simulink model "gm_DSBF"  (R2019b)
settings: Solver=FixedStepDiscrete  StartTime=0.0  StopTime=0.02  RelTol=1e-3
InitFcn:
  | sm_callback_init
StopFcn:
  | sm_callback_stop
undefined symbols (not defined in the file or in its folder): arraySize, arraySpacing, delayDataTypeFractionLength, delayDataTypeSign, delayDataTypeWordLength, mp, samplingRate, speedOfSound, upsampleFactor
libraries: hdlsllib x64, simulink x36, dspmlti4 x16, dsphdlfiltering x16
(part 1 of 5)
settings Model: Creator=Ross  LastModifiedBy=tyler
settings DataIOCC: ReturnWorkspaceOutputs=off
settings OptimizationCC: BlockReduction=off  ConditionallyExecuteInputs=off  DefaultParameterBehavior=Inlined
settings DebuggingCC: ReadBeforeWriteMsg=DisableAll  WriteAfterWriteMsg=DisableAll  WriteAfterReadMsg=DisableAll  AlgebraicLoopMsg=error  InheritedTsInSrcMsg=none  MultiTaskDSMMsg=none  SingleTaskRateTransMsg=error  PregeneratedLibrarySubsystemCodeDiagnostic=none  ArithmeticOperatorsInVariantConditions=warning
settings HardwareCC: ProdBitPerPointer=32  ProdBitPerSizeT=32  ProdBitPerPtrDiffT=32  ProdLargestAtomicFloat=None  ProdIntDivRoundTo=Undefined  ProdEndianess=Unspecified  ProdWordSize=32  ProdHWDeviceType=ASIC/FPGA->ASIC/FPGA  TargetBitPerPointer=64  TargetBitPerSizeT=64  TargetBitPerPtrDiffT=64  TargetLongLongMode=on  TargetIntDivRoundTo=Zero  TargetEndianess=LittleEndian  TargetWordSize=64  TargetHWDeviceType=Custom Processor->MATLAB Host Computer  ProdEqTarget=off
settings ModelReferenceCC: UpdateModelReferenceTargets=IfOutOfDate
settings SFSimCC: SFSimEcho=off  SimUseLocalCustomCode=off  CustomCodeUndefinedFunction=UseInterfaceOnly
settings RTWCC: RTWUseLocalCustomCode=off

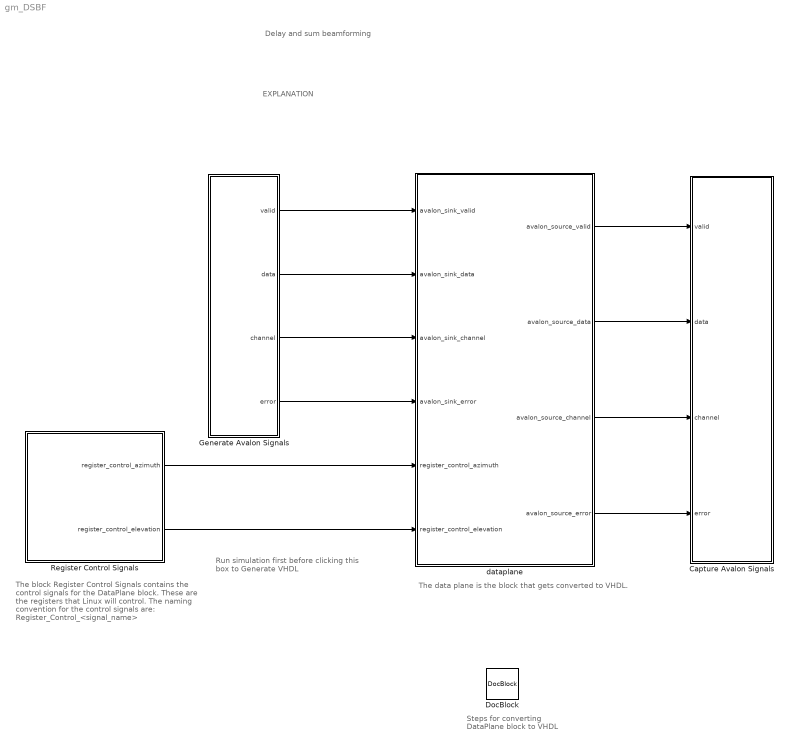
== system gm_DSBF ==
  note: The block Register Control Signals contains
      | the control signals for the DataPlane block.
      | These are the registers that Linux will control.
      | The naming convention for the control
      | signals are:  Register_Control_<signal_name>
  note: Run simulation first
      | before clicking this box to
      | Generate VHDL
  note: Delay and sum beamforming
  note: Steps for converting
      | DataPlane block
      | to VHDL
  note: EXPLANATION
  note: The data plane is the block that gets converted to VHDL.
  Capture Avalon Signals : Subsystem
  DocBlock : simulink/Model-Wide Utilities/DocBlock  DocumentType=HTML
  Generate Avalon Signals : Subsystem
  Register Control Signals : Subsystem
  dataplane : Subsystem  TreatAsAtomicUnit=on
  wires:
  Register Control Signals/2(register_control_elevation) -> dataplane/6(register_control_elevation)
  Register Control Signals/1(register_control_azimuth) -> dataplane/5(register_control_azimuth)
  dataplane/4(avalon_source_error) -> Capture Avalon Signals/4(error)
  dataplane/3(avalon_source_channel) -> Capture Avalon Signals/3(channel)
  dataplane/1(avalon_source_valid) -> Capture Avalon Signals/1(valid)
  dataplane/2(avalon_source_data) -> Capture Avalon Signals/2(data)
  Generate Avalon Signals/4(error) -> dataplane/4(avalon_sink_error)
  Generate Avalon Signals/3(channel) -> dataplane/3(avalon_sink_channel)
  Generate Avalon Signals/1(valid) -> dataplane/1(avalon_sink_valid)
  Generate Avalon Signals/2(data) -> dataplane/2(avalon_sink_data)

== system gm_DSBF/Capture Avalon Signals ==
  note: Note:  If these "To Workspace" variables show up under a variable called "out",
      | Open the Configure Logging... window (Simulation->Output->Configure Logging...)
      | and deselect the checkbox "Single simulation output:" found under the "Save to workspace or file" section.
  valid : Inport
  data : Inport  Port=2
  channel : Inport  Port=3
  error : Inport  Port=4
  To Workspace : ToWorkspace  VariableName=Avalon_Sink_Data  SaveFormat=Timeseries  SampleTime=-1
  To Workspace1 : ToWorkspace  VariableName=Avalon_Sink_Valid  SaveFormat=Timeseries  SampleTime=-1
  To Workspace2 : ToWorkspace  VariableName=Avalon_Sink_Channel  SaveFormat=Timeseries  SampleTime=-1
  To Workspace3 : ToWorkspace  VariableName=Avalon_Sink_Error  SaveFormat=Timeseries  SampleTime=-1
  wires:
  channel/1 -> To Workspace2/1
  error/1 -> To Workspace3/1
  valid/1 -> To Workspace1/1
  data/1 -> To Workspace/1

== system gm_DSBF/Generate Avalon Signals ==
  note: Avalon Streaming Sink Signals
      | Note: We are assuming a specific system clock frequency that these signals are being clock in at.
      | The interface needs to be regenerated if this system clock frequency changes. Change system clock frequency in InitFcn callback in Model Explorer.
      |
      | -- Avalon streaming slave interface (sink)
      | AD1939_DAC_data : in std_logic_vector(31 downto 0); -- W=32; F=28; Signed 2's Complement
      | AD1939_DAC_channel : in std_logic_vector(1 downto 0); -- Left <-> channel 0; Right <-> channel 1 (other two channels are ignored)
      | AD1939_DAC_valid : in std_logic; -- asserted when data is valid
      | AD1939_DAC_error : in std_logic_vector(1 downto 0) -- error channel is ignored, assumed to be error free at this point
      |
      | For more information on the data-channel-valid protocol, see chapter 5 in Intel's Avalon Interfaced Specification (p. 40) at https://www.intel.com/content/dam/www/programmable/us/en/pdfs/literature/manual/mnl_avalon_spec.pdf
  Avalon Source Channel : FromWorkspace  VariableName=mp.Avalon_Source_Channel  OutDataTypeStr=double  SampleTime=mp.Ts_system
  "Avalon Source Data " : FromWorkspace  VariableName=mp.Avalon_Source_Data  OutDataTypeStr=double  SampleTime=mp.Ts_system
  Avalon Source Error : FromWorkspace  VariableName=mp.Avalon_Source_Error  OutDataTypeStr=double  SampleTime=mp.Ts_system
  Avalon Source Valid : FromWorkspace  VariableName=mp.Avalon_Source_Valid  OutDataTypeStr=double  SampleTime=mp.Ts_system
  Data Type Conversion : DataTypeConversion  OutDataTypeStr=fixdt(1,mp.W_bits,mp.F_bits)
  Data Type Conversion1 : DataTypeConversion  OutDataTypeStr=fixdt(0,4,0)
  Data Type Conversion2 : DataTypeConversion  OutDataTypeStr=boolean
  Data Type Conversion3 : DataTypeConversion  OutDataTypeStr=fixdt(0,2,0)
  valid : Outport  VectorParamsAs1DForOutWhenUnconnected=off
  data : Outport  Port=2  VectorParamsAs1DForOutWhenUnconnected=off
  channel : Outport  Port=3  VectorParamsAs1DForOutWhenUnconnected=off
  error : Outport  Port=4  VectorParamsAs1DForOutWhenUnconnected=off
  wires:
  "Avalon Source Data "/1 -> Data Type Conversion/1
  Avalon Source Channel/1 -> Data Type Conversion1/1
  Data Type Conversion3/1 -> error/1
  Avalon Source Valid/1 -> Data Type Conversion2/1
  Data Type Conversion/1 -> data/1
  Avalon Source Error/1 -> Data Type Conversion3/1
  Data Type Conversion2/1 -> valid/1
  Data Type Conversion1/1 -> channel/1

== system gm_DSBF/Register Control Signals ==
  note: Control Signals that will be coming from Linux via
      | memory mapped registers need to have names
      | containing the prefix "register_control_"
      | (all lower case)
  Data Type Conversion1 : DataTypeConversion  OutDataTypeStr=mp.register(2).dataType
  Data Type Conversion2 : DataTypeConversion  OutDataTypeStr=mp.register(1).dataType
  Time Series Signal from Workspace 1 : FromWorkspace  VariableName=mp.register(1).timeseries  OutDataTypeStr=double  SampleTime=mp.Ts_system
  Time Series Signal from Workspace 2 : FromWorkspace  VariableName=mp.register(2).timeseries  OutDataTypeStr=double  SampleTime=mp.Ts_system
  register_control_azimuth : Outport  VectorParamsAs1DForOutWhenUnconnected=off
  register_control_elevation : Outport  Port=2  VectorParamsAs1DForOutWhenUnconnected=off
  wires:
  Data Type Conversion1/1 -> register_control_elevation/1
  Data Type Conversion2/1 -> register_control_azimuth/1
  Time Series Signal from Workspace 2/1 -> Data Type Conversion1/1
  Time Series Signal from Workspace 1/1 -> Data Type Conversion2/1

== system gm_DSBF/dataplane ==
  avalon_sink_valid : Inport  OutDataTypeStr=boolean  PortDimensions=1  SampleTime=1.01725260416667e-08
  avalon_sink_data : Inport  Port=2  OutDataTypeStr=fixdt(1, 32, 28)  PortDimensions=1  SampleTime=1.01725260416667e-08
  avalon_sink_channel : Inport  Port=3  OutDataTypeStr=fixdt(0, 4, 0)  PortDimensions=1  SampleTime=1.01725260416667e-08
  avalon_sink_error : Inport  Port=4  OutDataTypeStr=fixdt(0, 2, 0)  PortDimensions=1  SampleTime=1.01725260416667e-08
  register_control_azimuth : Inport  Port=5  OutDataTypeStr=fixdt(1, 16, 8)  PortDimensions=1  SampleTime=1.01725260416667e-08
  register_control_elevation : Inport  Port=6  OutDataTypeStr=fixdt(1, 16, 8)  PortDimensions=1  SampleTime=1.01725260416667e-08
  Avalon Data Processing : Subsystem
  Delay{,1..3} (4 alike) : Delay  DelayLength=double(1)  InitialCondition=0  SampleTime=1.01725260416667e-08
  compute projections : Subsystem
  compute_delays : Subsystem
  delayMatch : Delay  DelayLength=double(6144)  InitialCondition=0  SampleTime=1.01725260416667e-08
  delayMatch1 : Delay  DelayLength=double(6144)  InitialCondition=0  SampleTime=1.01725260416667e-08
  avalon_source_valid : Outport  VectorParamsAs1DForOutWhenUnconnected=off
  avalon_source_data : Outport  Port=2  VectorParamsAs1DForOutWhenUnconnected=off
  avalon_source_channel : Outport  Port=3  VectorParamsAs1DForOutWhenUnconnected=off
  avalon_source_error : Outport  Port=4  VectorParamsAs1DForOutWhenUnconnected=off
  wires:
  avalon_sink_valid/1 -> Avalon Data Processing/1(valid_in)
  avalon_sink_data/1 -> Avalon Data Processing/2(Sink_Data)
  avalon_sink_channel/1 -> Avalon Data Processing/3(Sink_Channel)
  delayMatch1/1 -> avalon_source_error/1
  register_control_azimuth/1 -> compute projections/1(azimuth)
  register_control_elevation/1 -> compute projections/2(elevation)
  Avalon Data Processing/1(Source_Data) -> avalon_source_data/1
  delayMatch/1 -> avalon_source_channel/1
  Avalon Data Processing/3(Source_Valid) -> avalon_source_valid/1
  Delay/1 -> compute_delays/3(sin_elevation)
  Delay1/1 -> compute_delays/2(cos_elevation)
  Delay2/1 -> compute_delays/1(sin_azimuth)
  Delay3/1 -> Avalon Data Processing/4(delays)
  compute projections/1(sin_azimuth) -> Delay2/1
  compute projections/2(cos_elevation) -> Delay1/1
  compute projections/3(sin_elevation) -> Delay/1
  compute_delays/1(delays) -> Delay3/1
  Avalon Data Processing/2(Source_Channel) -> delayMatch/1
  avalon_sink_error/1 -> delayMatch1/1

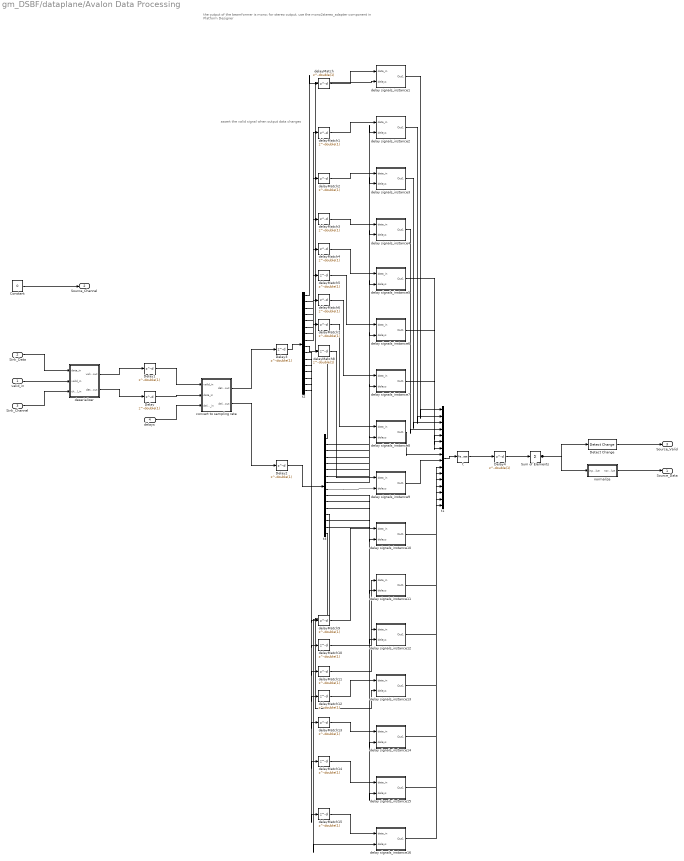
== system gm_DSBF/dataplane/Avalon Data Processing ==
  note: the output of the beamformer is mono; for stereo output, use the mono2stereo_adapter component in Platform Designer
  note: assert the valid signal when output data changes
  valid_in : Inport  OutDataTypeStr=boolean  PortDimensions=1  SampleTime=1.01725260416667e-08
  Sink_Data : Inport  Port=2  OutDataTypeStr=fixdt(1, 32, 28)  PortDimensions=1  SampleTime=1.01725260416667e-08
  Sink_Channel : Inport  Port=3  OutDataTypeStr=fixdt(0, 4, 0)  PortDimensions=1  SampleTime=1.01725260416667e-08
  delays : Inport  Port=4  OutDataTypeStr=fixdt(1, 12, 6)  PortDimensions=[16]  SampleTime=1.01725260416667e-08
  Constant : Constant  Value=0  OutDataTypeStr=fixdt(0, 1, 0)  SampleTime=-1
  Delay : Delay  DelayLength=double(1)  InitialCondition=0  SampleTime=1.01725260416667e-08
  Delay1 : Delay  DelayLength=double(1)  InitialCondition=0  SampleTime=1.01725260416667e-08
  Delay2 : Delay  DelayLength=double(1)  InitialCondition=0  SampleTime=2.08333333333333e-05
  Delay3 : Delay  DelayLength=double(1)  InitialCondition=0  SampleTime=2.08333333333333e-05
  Delay4 : Delay  DelayLength=double(1)  InitialCondition=0  SampleTime=1.01725260416667e-08
  Detect Change : simulink/Logic and Bit Operations/Detect Change  vinit=0  OutDataTypeStr=boolean
  Sum of Elements : Sum  Inputs=+  AccumDataTypeStr=fixdt(1, 36, 28)  OutDataTypeStr=fixdt(1, 36, 28)  SampleTime=1.01725260416667e-08
  convert to sampling rate : Subsystem
  delay signals_instance1 : Subsystem
  delay signals_instance10 : Subsystem
  delay signals_instance11 : Subsystem
  delay signals_instance12 : Subsystem
  delay signals_instance13 : Subsystem
  delay signals_instance14 : Subsystem
  delay signals_instance15 : Subsystem
  delay signals_instance16 : Subsystem
  delay signals_instance2 : Subsystem
  delay signals_instance3 : Subsystem
  delay signals_instance4 : Subsystem
  delay signals_instance5 : Subsystem
  delay signals_instance6 : Subsystem
  delay signals_instance7 : Subsystem
  delay signals_instance8 : Subsystem
  delay signals_instance9 : Subsystem
  delayMatch{,1..15} (16 alike) : Delay  DelayLength=double(1)  InitialCondition=0  SampleTime=2.08333333333333e-05
  deserializer : Subsystem
  normalize : Subsystem
  t : Reshape
  t1 : Concatenate  NumInputs=16
  t2 : Demux  Outputs=16
  t3 : Demux  Outputs=16
  Source_Data : Outport  InitialOutput=0  VectorParamsAs1DForOutWhenUnconnected=off
  Source_Channel : Outport  Port=2  InitialOutput=0  VectorParamsAs1DForOutWhenUnconnected=off
  Source_Valid : Outport  Port=3  InitialOutput=0  VectorParamsAs1DForOutWhenUnconnected=off
  wires:
  Delay/1 -> convert to sampling rate/2(data_in)
  Delay1/1 -> convert to sampling rate/1(valid_in)
  Delay2/1 -> t3/1
  Delay3/1 -> t2/1
  Delay4/1 -> Sum of Elements/1
  Detect Change/1 -> Source_Valid/1
  Sum of Elements/1 -> Detect Change/1, normalize/1(input_value)
  convert to sampling rate/1(data_out) -> Delay3/1
  convert to sampling rate/2(delays_out) -> Delay2/1
  t/1 -> Delay4/1
  deserializer/1(valid_out) -> Delay1/1
  deserializer/2(data_out) -> Delay/1
  delay signals_instance1/1(Out1) -> t1/1
  delay signals_instance2/1(Out1) -> t1/2
  delay signals_instance3/1(Out1) -> t1/3
  delay signals_instance4/1(Out1) -> t1/4
  delay signals_instance5/1(Out1) -> t1/5
  delay signals_instance6/1(Out1) -> t1/6
  delay signals_instance7/1(Out1) -> t1/7
  delay signals_instance8/1(Out1) -> t1/8
  delay signals_instance9/1(Out1) -> t1/9
  delay signals_instance10/1(Out1) -> t1/10
  delay signals_instance11/1(Out1) -> t1/11
  delay signals_instance12/1(Out1) -> t1/12
  delay signals_instance13/1(Out1) -> t1/13
  delay signals_instance14/1(Out1) -> t1/14
  delay signals_instance15/1(Out1) -> t1/15
  delay signals_instance16/1(Out1) -> t1/16
  normalize/1(normalized_value) -> Source_Data/1
  Constant/1 -> Source_Channel/1
  delayMatch/1 -> delay signals_instance1/1(data_in)
  delayMatch1/1 -> delay signals_instance2/1(data_in)
  delayMatch2/1 -> delay signals_instance3/1(data_in)
  delayMatch3/1 -> delay signals_instance4/1(data_in)
  delayMatch4/1 -> delay signals_instance5/1(data_in)
  delayMatch5/1 -> delay signals_instance6/1(data_in)
  delayMatch6/1 -> delay signals_instance7/1(data_in)
  delayMatch7/1 -> delay signals_instance8/1(data_in)
  delayMatch8/1 -> delay signals_instance9/1(data_in)
  delayMatch9/1 -> delay signals_instance10/1(data_in)
  delayMatch10/1 -> delay signals_instance11/1(data_in)
  delayMatch11/1 -> delay signals_instance12/1(data_in)
  delayMatch12/1 -> delay signals_instance13/1(data_in)
  delayMatch13/1 -> delay signals_instance14/1(data_in)
  delayMatch14/1 -> delay signals_instance15/1(data_in)
  delayMatch15/1 -> delay signals_instance16/1(data_in)
  t3/1 -> delay signals_instance1/2(delays)
  t3/2 -> delay signals_instance2/2(delays)
  t3/3 -> delay signals_instance3/2(delays)
  t3/4 -> delay signals_instance4/2(delays)
  t3/5 -> delay signals_instance5/2(delays)
  t3/6 -> delay signals_instance6/2(delays)
  t3/7 -> delay signals_instance7/2(delays)
  t3/8 -> delay signals_instance8/2(delays)
  t3/9 -> delay signals_instance9/2(delays)
  t3/10 -> delay signals_instance10/2(delays)
  t3/11 -> delay signals_instance11/2(delays)
  t3/12 -> delay signals_instance12/2(delays)
  t3/13 -> delay signals_instance13/2(delays)
  t3/14 -> delay signals_instance14/2(delays)
  t3/15 -> delay signals_instance15/2(delays)
  t3/16 -> delay signals_instance16/2(delays)
  t1/1 -> t/1
  valid_in/1 -> deserializer/2(valid_in)
  Sink_Data/1 -> deserializer/1(data_in)
  Sink_Channel/1 -> deserializer/3(channel_in)
  delays/1 -> convert to sampling rate/3(delays_in)
  t2/1 -> delayMatch/1
  t2/2 -> delayMatch1/1
  t2/3 -> delayMatch2/1
  t2/4 -> delayMatch3/1
  t2/5 -> delayMatch4/1
  t2/6 -> delayMatch5/1
  t2/7 -> delayMatch6/1
  t2/8 -> delayMatch7/1
  t2/9 -> delayMatch8/1
  t2/10 -> delayMatch9/1
  t2/11 -> delayMatch10/1
  t2/12 -> delayMatch11/1
  t2/13 -> delayMatch12/1
  t2/14 -> delayMatch13/1
  t2/15 -> delayMatch14/1
  t2/16 -> delayMatch15/1

== system gm_DSBF/dataplane/compute projections ==
  azimuth : Inport  OutDataTypeStr=fixdt(1, 16, 8)  PortDimensions=1  SampleTime=1.01725260416667e-08
  elevation : Inport  Port=2  OutDataTypeStr=fixdt(1, 16, 8)  PortDimensions=1  SampleTime=1.01725260416667e-08
  compute cosine : Subsystem
  compute sine : Subsystem
  compute sine1 : Subsystem
  sin_azimuth : Outport
  cos_elevation : Outport  Port=2
  sin_elevation : Outport  Port=3
  wires:
  compute cosine/1(Out1) -> cos_elevation/1
  compute sine/1(output_value) -> sin_azimuth/1
  compute sine1/1(output_value) -> sin_elevation/1
  azimuth/1 -> compute sine/1(angle)
  elevation/1 -> compute sine1/1(angle), compute cosine/1(angle)

== system gm_DSBF/dataplane/compute_delays ==
  sin_azimuth : Inport  OutDataTypeStr=fixdt(1, 16, 14)  PortDimensions=1  SampleTime=1.01725260416667e-08
  cos_elevation : Inport  Port=2  OutDataTypeStr=fixdt(1, 16, 14)  PortDimensions=1  SampleTime=1.01725260416667e-08
  sin_elevation : Inport  Port=3  OutDataTypeStr=fixdt(1, 16, 14)  PortDimensions=1  SampleTime=1.01725260416667e-08
  compute_delays : MATLAB Function  TreatAsAtomicUnit=on
  delayMatch : Delay  DelayLength=double(4)  InitialCondition=0  SampleTime=1.01725260416667e-08
  delays : Outport  VectorParamsAs1DForOutWhenUnconnected=off
  wires:
  delayMatch/1 -> compute_delays/2(cos_elevation)
  compute_delays/1(delays) -> delays/1
  sin_azimuth/1 -> compute_delays/1(sin_azimuth)
  cos_elevation/1 -> delayMatch/1
  sin_elevation/1 -> compute_delays/3(sin_elevation)

== system gm_DSBF/dataplane/Avalon Data Processing/convert to sampling rate ==
  note: sample and data on the valid pulse to make sure we are only using valid data
  valid_in : Inport  OutDataTypeStr=boolean  PortDimensions=1  SampleTime=1.01725260416667e-08
  data_in : Inport  Port=2  OutDataTypeStr=fixdt(1, 32, 28)  PortDimensions=[16]  SampleTime=1.01725260416667e-08
  delays_in : Inport  Port=3  OutDataTypeStr=fixdt(1, 12, 6)  PortDimensions=[16]  SampleTime=1.01725260416667e-08
  PipelineRegister : Delay  DelayLength=double(1)  InitialCondition=0  SampleTime=2.08333333333333e-05
  PipelineRegister1 : Delay  DelayLength=double(1)  InitialCondition=0  SampleTime=2.08333333333333e-05
  Rate Transition1 : RateTransition  InitialCondition=double(0)  OutPortSampleTimeOpt=Multiple of input port sample time  OutPortSampleTimeMultiple=2048
  Rate Transition2 : DownSample  N=double(2048)  phase=double(4)  RateOptions=Allow multirate processing
  Sample and Hold : Subsystem  mask(Sample and Hold){trig=Rising edge, initCond=double(0), latchinput=off}
      mask prompts: trig "Trigger type:"; initCond "Initial condition:"; latchinput "Latch (buffer) input"
      mask help: Sample and hold the input signal. If Latch (buffer) input is selected, then this block produces the value of the input from the previous time step.
      mask init:
      | switch trig
      | case 1, s='rising';
      | case 2, s='falling';
      | case 3, s='either';
      | end
      | set_param([gcb '/Trigger'],'triggertype',s);
      | if (latchinput == 1)
      | 	set_param([gcb '/In'],'latchinput','on');
      | else
      | 	set_param([gcb '/In'],'latchinput','off');
      | end
      mask Help: eval('blocksethelp');
      mask TypeOptions trig: Rising edge | Falling edge | Either edge
      mask Display: disp('S/H')
  Sample and Hold1 : Subsystem  mask(Sample and Hold){trig=Rising edge, initCond=double(0), latchinput=off}
      mask prompts: trig "Trigger type:"; initCond "Initial condition:"; latchinput "Latch (buffer) input"
      mask help: Sample and hold the input signal. If Latch (buffer) input is selected, then this block produces the value of the input from the previous time step.
      mask init: same as gm_DSBF/dataplane/Avalon Data Processing/convert to sampling rate/Sample and Hold
      mask Help: eval('blocksethelp');
      mask TypeOptions trig: Rising edge | Falling edge | Either edge
      mask Display: disp('S/H')
  delayMatch : Delay  DelayLength=double(4)  InitialCondition=0  SampleTime=1.01725260416667e-08
  data_out : Outport
  delays_out : Outport  Port=2
  wires:
  delayMatch/1 -> Sample and Hold1/Trigger
  PipelineRegister/1 -> data_out/1
  PipelineRegister1/1 -> delays_out/1
  Sample and Hold/1(" ") -> Rate Transition1/1
  valid_in/1 -> delayMatch/1, Sample and Hold/Trigger
  data_in/1 -> Sample and Hold/1(In)
  delays_in/1 -> Sample and Hold1/1(In)
  Sample and Hold1/1(" ") -> Rate Transition2/1
  Rate Transition1/1 -> PipelineRegister/1
  Rate Transition2/1 -> PipelineRegister1/1

== system gm_DSBF/dataplane/Avalon Data Processing/delay signals_instance1 ==
  data_in : Inport  OutDataTypeStr=fixdt(1, 32, 28)  PortDimensions=1  SampleTime=2.08333333333333e-05
  delays : Inport  Port=2  OutDataTypeStr=fixdt(1, 12, 6)  PortDimensions=1  SampleTime=2.08333333333333e-05
  delay signal : Subsystem
  Out1 : Outport  VectorParamsAs1DForOutWhenUnconnected=off
  wires:
  delay signal/1(data_out) -> Out1/1
  data_in/1 -> delay signal/1(data_in)
  delays/1 -> delay signal/2(delay)

== system gm_DSBF/dataplane/Avalon Data Processing/delay signals_instance10 ==
  data_in : Inport  OutDataTypeStr=fixdt(1, 32, 28)  PortDimensions=1  SampleTime=2.08333333333333e-05
  delays : Inport  Port=2  OutDataTypeStr=fixdt(1, 12, 6)  PortDimensions=1  SampleTime=2.08333333333333e-05
  delay signal : Subsystem
  Out1 : Outport  VectorParamsAs1DForOutWhenUnconnected=off
  wires:
  delays/1 -> delay signal/2(delay)
  data_in/1 -> delay signal/1(data_in)
  delay signal/1(data_out) -> Out1/1

== system gm_DSBF/dataplane/Avalon Data Processing/delay signals_instance11 ==
  data_in : Inport  OutDataTypeStr=fixdt(1, 32, 28)  PortDimensions=1  SampleTime=2.08333333333333e-05
  delays : Inport  Port=2  OutDataTypeStr=fixdt(1, 12, 6)  PortDimensions=1  SampleTime=2.08333333333333e-05
  delay signal : Subsystem
  Out1 : Outport  VectorParamsAs1DForOutWhenUnconnected=off
  wires:
  delays/1 -> delay signal/2(delay)
  data_in/1 -> delay signal/1(data_in)
  delay signal/1(data_out) -> Out1/1

== system gm_DSBF/dataplane/Avalon Data Processing/delay signals_instance12 ==
  data_in : Inport  OutDataTypeStr=fixdt(1, 32, 28)  PortDimensions=1  SampleTime=2.08333333333333e-05
  delays : Inport  Port=2  OutDataTypeStr=fixdt(1, 12, 6)  PortDimensions=1  SampleTime=2.08333333333333e-05
  delay signal : Subsystem
  Out1 : Outport  VectorParamsAs1DForOutWhenUnconnected=off
  wires:
  delays/1 -> delay signal/2(delay)
  data_in/1 -> delay signal/1(data_in)
  delay signal/1(data_out) -> Out1/1

== system gm_DSBF/dataplane/Avalon Data Processing/delay signals_instance13 ==
  data_in : Inport  OutDataTypeStr=fixdt(1, 32, 28)  PortDimensions=1  SampleTime=2.08333333333333e-05
  delays : Inport  Port=2  OutDataTypeStr=fixdt(1, 12, 6)  PortDimensions=1  SampleTime=2.08333333333333e-05
  delay signal : Subsystem
  Out1 : Outport  VectorParamsAs1DForOutWhenUnconnected=off
  wires:
  delays/1 -> delay signal/2(delay)
  data_in/1 -> delay signal/1(data_in)
  delay signal/1(data_out) -> Out1/1

== system gm_DSBF/dataplane/Avalon Data Processing/delay signals_instance14 ==
  data_in : Inport  OutDataTypeStr=fixdt(1, 32, 28)  PortDimensions=1  SampleTime=2.08333333333333e-05
  delays : Inport  Port=2  OutDataTypeStr=fixdt(1, 12, 6)  PortDimensions=1  SampleTime=2.08333333333333e-05
  delay signal : Subsystem
  Out1 : Outport  VectorParamsAs1DForOutWhenUnconnected=off
  wires:
  delays/1 -> delay signal/2(delay)
  data_in/1 -> delay signal/1(data_in)
  delay signal/1(data_out) -> Out1/1

== system gm_DSBF/dataplane/Avalon Data Processing/delay signals_instance15 ==
  data_in : Inport  OutDataTypeStr=fixdt(1, 32, 28)  PortDimensions=1  SampleTime=2.08333333333333e-05
  delays : Inport  Port=2  OutDataTypeStr=fixdt(1, 12, 6)  PortDimensions=1  SampleTime=2.08333333333333e-05
  delay signal : Subsystem
  Out1 : Outport  VectorParamsAs1DForOutWhenUnconnected=off
  wires:
  delays/1 -> delay signal/2(delay)
  data_in/1 -> delay signal/1(data_in)
  delay signal/1(data_out) -> Out1/1

== system gm_DSBF/dataplane/Avalon Data Processing/delay signals_instance16 ==
  data_in : Inport  OutDataTypeStr=fixdt(1, 32, 28)  PortDimensions=1  SampleTime=2.08333333333333e-05
  delays : Inport  Port=2  OutDataTypeStr=fixdt(1, 12, 6)  PortDimensions=1  SampleTime=2.08333333333333e-05
  delay signal : Subsystem
  Out1 : Outport  VectorParamsAs1DForOutWhenUnconnected=off
  wires:
  delays/1 -> delay signal/2(delay)
  data_in/1 -> delay signal/1(data_in)
  delay signal/1(data_out) -> Out1/1

== system gm_DSBF/dataplane/Avalon Data Processing/delay signals_instance2 ==
  data_in : Inport  OutDataTypeStr=fixdt(1, 32, 28)  PortDimensions=1  SampleTime=2.08333333333333e-05
  delays : Inport  Port=2  OutDataTypeStr=fixdt(1, 12, 6)  PortDimensions=1  SampleTime=2.08333333333333e-05
  delay signal : Subsystem
  Out1 : Outport  VectorParamsAs1DForOutWhenUnconnected=off
  wires:
  delays/1 -> delay signal/2(delay)
  data_in/1 -> delay signal/1(data_in)
  delay signal/1(data_out) -> Out1/1

== system gm_DSBF/dataplane/Avalon Data Processing/delay signals_instance3 ==
  data_in : Inport  OutDataTypeStr=fixdt(1, 32, 28)  PortDimensions=1  SampleTime=2.08333333333333e-05
  delays : Inport  Port=2  OutDataTypeStr=fixdt(1, 12, 6)  PortDimensions=1  SampleTime=2.08333333333333e-05
  delay signal : Subsystem
  Out1 : Outport  VectorParamsAs1DForOutWhenUnconnected=off
  wires:
  delays/1 -> delay signal/2(delay)
  data_in/1 -> delay signal/1(data_in)
  delay signal/1(data_out) -> Out1/1

== system gm_DSBF/dataplane/Avalon Data Processing/delay signals_instance4 ==
  data_in : Inport  OutDataTypeStr=fixdt(1, 32, 28)  PortDimensions=1  SampleTime=2.08333333333333e-05
  delays : Inport  Port=2  OutDataTypeStr=fixdt(1, 12, 6)  PortDimensions=1  SampleTime=2.08333333333333e-05
  delay signal : Subsystem
  Out1 : Outport  VectorParamsAs1DForOutWhenUnconnected=off
  wires:
  delays/1 -> delay signal/2(delay)
  data_in/1 -> delay signal/1(data_in)
  delay signal/1(data_out) -> Out1/1

== system gm_DSBF/dataplane/Avalon Data Processing/delay signals_instance5 ==
  data_in : Inport  OutDataTypeStr=fixdt(1, 32, 28)  PortDimensions=1  SampleTime=2.08333333333333e-05
  delays : Inport  Port=2  OutDataTypeStr=fixdt(1, 12, 6)  PortDimensions=1  SampleTime=2.08333333333333e-05
  delay signal : Subsystem
  Out1 : Outport  VectorParamsAs1DForOutWhenUnconnected=off
  wires:
  delays/1 -> delay signal/2(delay)
  data_in/1 -> delay signal/1(data_in)
  delay signal/1(data_out) -> Out1/1

== system gm_DSBF/dataplane/Avalon Data Processing/delay signals_instance6 ==
  data_in : Inport  OutDataTypeStr=fixdt(1, 32, 28)  PortDimensions=1  SampleTime=2.08333333333333e-05
  delays : Inport  Port=2  OutDataTypeStr=fixdt(1, 12, 6)  PortDimensions=1  SampleTime=2.08333333333333e-05
  delay signal : Subsystem
  Out1 : Outport  VectorParamsAs1DForOutWhenUnconnected=off
  wires:
  delays/1 -> delay signal/2(delay)
  data_in/1 -> delay signal/1(data_in)
  delay signal/1(data_out) -> Out1/1

== system gm_DSBF/dataplane/Avalon Data Processing/delay signals_instance7 ==
  data_in : Inport  OutDataTypeStr=fixdt(1, 32, 28)  PortDimensions=1  SampleTime=2.08333333333333e-05
  delays : Inport  Port=2  OutDataTypeStr=fixdt(1, 12, 6)  PortDimensions=1  SampleTime=2.08333333333333e-05
  delay signal : Subsystem
  Out1 : Outport  VectorParamsAs1DForOutWhenUnconnected=off
  wires:
  delays/1 -> delay signal/2(delay)
  data_in/1 -> delay signal/1(data_in)
  delay signal/1(data_out) -> Out1/1

== system gm_DSBF/dataplane/Avalon Data Processing/delay signals_instance8 ==
  data_in : Inport  OutDataTypeStr=fixdt(1, 32, 28)  PortDimensions=1  SampleTime=2.08333333333333e-05
  delays : Inport  Port=2  OutDataTypeStr=fixdt(1, 12, 6)  PortDimensions=1  SampleTime=2.08333333333333e-05
  delay signal : Subsystem
  Out1 : Outport  VectorParamsAs1DForOutWhenUnconnected=off
  wires:
  delays/1 -> delay signal/2(delay)
  data_in/1 -> delay signal/1(data_in)
  delay signal/1(data_out) -> Out1/1

== system gm_DSBF/dataplane/Avalon Data Processing/delay signals_instance9 ==
  data_in : Inport  OutDataTypeStr=fixdt(1, 32, 28)  PortDimensions=1  SampleTime=2.08333333333333e-05
  delays : Inport  Port=2  OutDataTypeStr=fixdt(1, 12, 6)  PortDimensions=1  SampleTime=2.08333333333333e-05
  delay signal : Subsystem
  Out1 : Outport  VectorParamsAs1DForOutWhenUnconnected=off
  wires:
  delays/1 -> delay signal/2(delay)
  data_in/1 -> delay signal/1(data_in)
  delay signal/1(data_out) -> Out1/1

== system gm_DSBF/dataplane/Avalon Data Processing/deserializer ==
  data_in : Inport  OutDataTypeStr=fixdt(1, 32, 28)  PortDimensions=1  SampleTime=1.01725260416667e-08
  valid_in : Inport  Port=2  OutDataTypeStr=boolean  PortDimensions=1  SampleTime=1.01725260416667e-08
  channel_in : Inport  Port=3  OutDataTypeStr=fixdt(0, 4, 0)  PortDimensions=1  SampleTime=1.01725260416667e-08
  deserializer : MATLAB Function  TreatAsAtomicUnit=on
  valid_out : Outport
  data_out : Outport  Port=2  VectorParamsAs1DForOutWhenUnconnected=off
  wires:
  deserializer/1(valid_out) -> valid_out/1
  deserializer/2(data_out) -> data_out/1
  data_in/1 -> deserializer/1(data_in)
  valid_in/1 -> deserializer/2(valid_in)
  channel_in/1 -> deserializer/3(channel_in)

== system gm_DSBF/dataplane/Avalon Data Processing/normalize ==
  input_value : Inport  OutDataTypeStr=fixdt(1, 36, 28)  PortDimensions=1  SampleTime=1.01725260416667e-08
  Data Type Conversion : DataTypeConversion  OutDataTypeStr=fixdt(1, mp.W_bits, mp.F_bits)
  normalize_shift : Subsystem
  normalized_value : Outport
  wires:
  Data Type Conversion/1 -> normalized_value/1
  normalize_shift/1(normalized) -> Data Type Conversion/1
  input_value/1 -> normalize_shift/1(input)

== system gm_DSBF/dataplane/compute projections/compute cosine ==
  angle : Inport  OutDataTypeStr=fixdt(1, 16, 8)  PortDimensions=1  SampleTime=1.01725260416667e-08
  Abs : Abs
  cos LUT : Subsystem
  Out1 : Outport
  wires:
  Abs/1 -> cos LUT/1(In1)
  cos LUT/1(Out1) -> Out1/1
  angle/1 -> Abs/1

== system gm_DSBF/dataplane/compute projections/compute sine ==
  angle : Inport  OutDataTypeStr=fixdt(1, 16, 8)  PortDimensions=1  SampleTime=1.01725260416667e-08
  Compare To Zero : simulink/Logic and Bit Operations/Compare To Constant  relop=>  const=double(0)  OutDataTypeStr=boolean
  Constant : Constant  Value=-1  OutDataTypeStr=fixdt(1, 16, 8)  SampleTime=-1
  Constant1 : Constant  Value=-1  OutDataTypeStr=fixdt(1, 16, 14)  SampleTime=-1
  HwModeRegister{,1..3} (4 alike) : Delay  DelayLength=double(1)  InitialCondition=0  SampleTime=1.01725260416667e-08
  PipelineRegister : Delay  DelayLength=double(1)  InitialCondition=0  SampleTime=1.01725260416667e-08
  PipelineRegister1 : Delay  DelayLength=double(1)  InitialCondition=0  SampleTime=1.01725260416667e-08
  Product : Product  Inputs=**  OutDataTypeStr=fixdt(1, 16, 8)  SampleTime=1.01725260416667e-08
  Product1 : Product  Inputs=**  OutDataTypeStr=fixdt(1, 16, 14)  SampleTime=1.01725260416667e-08
  Switch : Switch  Criteria=u2 ~= 0  Threshold=double(0)  OutDataTypeStr=fixdt(1, 16, 8)  SampleTime=1.01725260416667e-08
  Switch1 : Switch  Criteria=u2 ~= 0  Threshold=double(0)  OutDataTypeStr=fixdt(1, 16, 14)  SampleTime=1.01725260416667e-08
  delayMatch : Delay  DelayLength=double(2)  InitialCondition=0  SampleTime=1.01725260416667e-08
  delayMatch1 : Delay  DelayLength=double(2)  InitialCondition=0  SampleTime=1.01725260416667e-08
  delayMatch2 : Delay  DelayLength=double(2)  InitialCondition=0  SampleTime=1.01725260416667e-08
  delayMatch3 : Delay  DelayLength=double(4)  InitialCondition=0  SampleTime=1.01725260416667e-08
  sin LUT : Subsystem
  output_value : Outport
  wires:
  delayMatch/1 -> Switch/1
  delayMatch1/1 -> Switch/2
  Constant/1 -> HwModeRegister1/1
  Constant1/1 -> HwModeRegister3/1
  PipelineRegister/1 -> Switch/3
  PipelineRegister1/1 -> Switch1/3
  Switch/1 -> sin LUT/1(angle)
  Switch1/1 -> output_value/1
  delayMatch2/1 -> Switch1/1
  angle/1 -> delayMatch/1, Compare To Zero/1, HwModeRegister/1
  delayMatch3/1 -> Switch1/2
  sin LUT/1(sin_angle) -> delayMatch2/1, HwModeRegister2/1
  Compare To Zero/1 -> delayMatch3/1, delayMatch1/1
  Product/1 -> PipelineRegister/1
  HwModeRegister/1 -> Product/1
  HwModeRegister1/1 -> Product/2
  Product1/1 -> PipelineRegister1/1
  HwModeRegister2/1 -> Product1/1
  HwModeRegister3/1 -> Product1/2

== system gm_DSBF/dataplane/compute projections/compute sine1 ==
  angle : Inport  OutDataTypeStr=fixdt(1, 16, 8)  PortDimensions=1  SampleTime=1.01725260416667e-08
  Compare To Zero : simulink/Logic and Bit Operations/Compare To Constant  relop=>  const=double(0)  OutDataTypeStr=boolean
  Constant : Constant  Value=-1  OutDataTypeStr=fixdt(1, 16, 8)  SampleTime=-1
  Constant1 : Constant  Value=-1  OutDataTypeStr=fixdt(1, 16, 14)  SampleTime=-1
  HwModeRegister{,1..3} (4 alike) : Delay  DelayLength=double(1)  InitialCondition=0  SampleTime=1.01725260416667e-08
  PipelineRegister : Delay  DelayLength=double(1)  InitialCondition=0  SampleTime=1.01725260416667e-08
  PipelineRegister1 : Delay  DelayLength=double(1)  InitialCondition=0  SampleTime=1.01725260416667e-08
  Product : Product  Inputs=**  OutDataTypeStr=fixdt(1, 16, 8)  SampleTime=1.01725260416667e-08
  Product1 : Product  Inputs=**  OutDataTypeStr=fixdt(1, 16, 14)  SampleTime=1.01725260416667e-08
  Switch : Switch  Criteria=u2 ~= 0  Threshold=double(0)  OutDataTypeStr=fixdt(1, 16, 8)  SampleTime=1.01725260416667e-08
  Switch1 : Switch  Criteria=u2 ~= 0  Threshold=double(0)  OutDataTypeStr=fixdt(1, 16, 14)  SampleTime=1.01725260416667e-08
  delayMatch : Delay  DelayLength=double(2)  InitialCondition=0  SampleTime=1.01725260416667e-08
  delayMatch1 : Delay  DelayLength=double(2)  InitialCondition=0  SampleTime=1.01725260416667e-08
  delayMatch2 : Delay  DelayLength=double(2)  InitialCondition=0  SampleTime=1.01725260416667e-08
  delayMatch3 : Delay  DelayLength=double(4)  InitialCondition=0  SampleTime=1.01725260416667e-08
  sin LUT : Subsystem
  output_value : Outport
  wires:
  delayMatch/1 -> Switch/1
  delayMatch1/1 -> Switch/2
  Constant/1 -> HwModeRegister1/1
  Constant1/1 -> HwModeRegister3/1
  PipelineRegister/1 -> Switch/3
  PipelineRegister1/1 -> Switch1/3
  Switch/1 -> sin LUT/1(angle)
  Switch1/1 -> output_value/1
  delayMatch2/1 -> Switch1/1
  angle/1 -> delayMatch/1, Compare To Zero/1, HwModeRegister/1
  delayMatch3/1 -> Switch1/2
  sin LUT/1(sin_angle) -> delayMatch2/1, HwModeRegister2/1
  Compare To Zero/1 -> delayMatch3/1, delayMatch1/1
  Product/1 -> PipelineRegister/1
  HwModeRegister/1 -> Product/1
  HwModeRegister1/1 -> Product/2
  Product1/1 -> PipelineRegister1/1
  HwModeRegister2/1 -> Product1/1
  HwModeRegister3/1 -> Product1/2

== system gm_DSBF/dataplane/Avalon Data Processing/convert to sampling rate/Sample and Hold ==
  note: Trigger
  In : Inport  OutDataTypeStr=fixdt(1, 32, 28)  PortDimensions=[16]
  Trigger : TriggerPort  VariantControl=(inherit)  OutDataTypeStr=boolean
  " " : Outport  InitialOutput=0
  wires:
  In/1 -> " "/1

== system gm_DSBF/dataplane/Avalon Data Processing/convert to sampling rate/Sample and Hold1 ==
  note: Trigger
  In : Inport  OutDataTypeStr=fixdt(1, 12, 6)  PortDimensions=[16]
  Trigger : TriggerPort  VariantControl=(inherit)  OutDataTypeStr=boolean
  " " : Outport  InitialOutput=0
  wires:
  In/1 -> " "/1

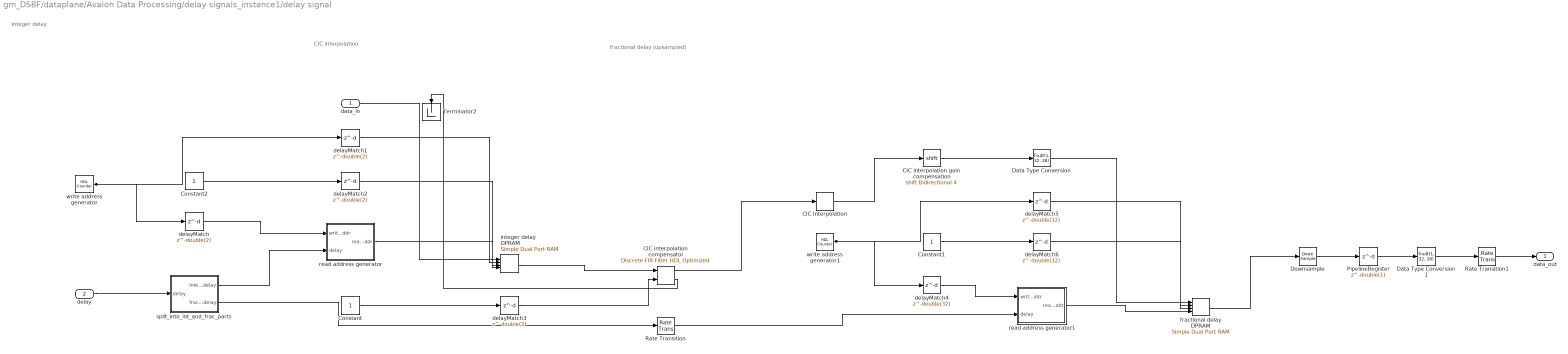
== system gm_DSBF/dataplane/Avalon Data Processing/delay signals_instance1/delay signal ==
  note: fractional delay (upsampled)
  note: Integer delay
  note: CIC interpolation
  data_in : Inport  OutDataTypeStr=fixdt(1, 32, 28)  PortDimensions=1  SampleTime=2.08333333333333e-05
  delay : Inport  Port=2  OutDataTypeStr=fixdt(1, 12, 6)  PortDimensions=1  SampleTime=2.08333333333333e-05
  CIC Interpolation : dspmlti4/CIC Interpolation  filtFrom=Filter object  filtobj=mp.cicInterpolator  ftype=Interpolator  R=mp.upsampleFactor  M=1  N=2  filterInternals=Full precision  BPS=[16 16 16 16]  FLPS=0  outputWordLength=32  outputFracLength=0  launchFVT=off  framing=Allow multirate processing  OutputFrames=off
      settings: SourceProductName=DSP System Toolbox  SourceProductBaseCode=DS
  CIC interpolation compensator : dsphdlfiltering/Discrete FIR Filter HDL Optimized  NumeratorSource=Property  Numerator=mp.cicInterpolatorCompensator.coeffs.Numerator  NumeratorPrototype=[]  FilterStructure=Direct form systolic  SerializationOption=Maximum number of multipliers  NumberOfCycles=2  NumberOfMultipliers=4  SimulateUsing=Code generation  roundingMode=Floor  overflowMode=off  CoefficientsDataTypeStr=fixdt(1,16)  CoefficientsMin=[]  CoefficientsMax=[]  OutputDataTypeStr=Inherit: Same word length as input  OutputMin=[]  OutputMax=[]  ResetInputPort=off  HDLGlobalReset=off
      settings: SourceProductName=DSP System Toolbox  SourceProductBaseCode=DS
  CIC interpolation gain compensation : ArithShift  BitShiftNumber=4  BinPtShiftNumber=double(0)
  Constant : Constant  OutDataTypeStr=boolean  SampleTime=-1
  Constant1 : Constant  OutDataTypeStr=boolean  SampleTime=-1
  Constant2 : Constant  OutDataTypeStr=boolean  SampleTime=-1
  Data Type Conversion : DataTypeConversion  OutDataTypeStr=fixdt(1, 32, 28)  SampleTime=1.30208333333333e-06
  Data Type Conversion1 : DataTypeConversion  OutDataTypeStr=fixdt(1, 32, 28)  SampleTime=2.08333333333333e-05
  Downsample : DownSample  N=double(16)  phase=double(0)  RateOptions=Allow multirate processing
  PipelineRegister : Delay  DelayLength=double(1)  InitialCondition=0  SampleTime=2.08333333333333e-05
  Rate Transition : RateTransition  InitialCondition=double(0)  OutPortSampleTimeOpt=Multiple of input port sample time  OutPortSampleTimeMultiple=1/16
  Rate Transition1 : RateTransition  InitialCondition=double(0)  OutPortSampleTimeOpt=Multiple of input port sample time  OutPortSampleTimeMultiple=1/2048
  Terminator2 : Terminator
  delayMatch{,1..3} (4 alike) : Delay  DelayLength=double(2)  InitialCondition=0  SampleTime=2.08333333333333e-05
  delayMatch4 : Delay  DelayLength=double(32)  InitialCondition=0  SampleTime=1.30208333333333e-06
  delayMatch5 : Delay  DelayLength=double(32)  InitialCondition=0  SampleTime=1.30208333333333e-06
  delayMatch6 : Delay  DelayLength=double(32)  InitialCondition=0  SampleTime=1.30208333333333e-06
  fractional delay DPRAM : hdlsllib/HDL RAMs/Simple Dual Port RAM  ram_size=mp.fractionalDelayAddrSize
      settings: SourceProductName=Simulink  SourceProductBaseCode=SL
  integer delay DPRAM : hdlsllib/HDL RAMs/Simple Dual Port RAM  ram_size=mp.integerDelayAddrSize
      settings: SourceProductName=Simulink  SourceProductBaseCode=SL
  read address generator : Subsystem
  read address generator1 : Subsystem
  split_into_int_and_frac_parts : Subsystem
  write address generator : hdlsllib/Sources/HDL Counter  CountType=Count limited  CountInit=double(0)  CountStep=double(1)  CountMax=double(63)  CountFromType=Initial value  CountFrom=double(0)  CountResetPort=off  CountLoadPort=off  CountEnbPort=off  CountDirPort=off  CountDataType=Unsigned  CountWordLen=6  CountFracLen=0  CountSampTime=2.08333333333333e-05
      settings: SourceProductName=Simulink
  write address generator1 : hdlsllib/Sources/HDL Counter  CountType=Count limited  CountInit=double(0)  CountStep=double(1)  CountMax=double(63)  CountFromType=Initial value  CountFrom=double(0)  CountResetPort=off  CountLoadPort=off  CountEnbPort=off  CountDirPort=off  CountDataType=Unsigned  CountWordLen=6  CountFracLen=0  CountSampTime=1.30208333333333e-06
      settings: SourceProductName=Simulink
  data_out : Outport  VectorParamsAs1DForOutWhenUnconnected=off
  wires:
  delayMatch4/1 -> read address generator1/1(write_addr)
  delayMatch/1 -> read address generator/1(write_addr)
  integer delay DPRAM/1 -> CIC interpolation compensator/1
  fractional delay DPRAM/1 -> Downsample/1
  Rate Transition1/1 -> data_out/1
  Rate Transition/1 -> read address generator1/2(delay)
  PipelineRegister/1 -> Data Type Conversion1/1
  CIC interpolation compensator/1 -> CIC Interpolation/1
  CIC interpolation compensator/2 -> Terminator2/1
  CIC Interpolation/1 -> CIC interpolation gain compensation/1
  read address generator1/1(read_addr) -> fractional delay DPRAM/4
  read address generator/1(read_addr) -> integer delay DPRAM/4
  split_into_int_and_frac_parts/2(fractional_delay) -> Rate Transition/1
  Data Type Conversion1/1 -> Rate Transition1/1
  Data Type Conversion/1 -> fractional delay DPRAM/1
  delayMatch2/1 -> integer delay DPRAM/3
  delayMatch6/1 -> fractional delay DPRAM/3
  delayMatch3/1 -> CIC interpolation compensator/2
  data_in/1 -> integer delay DPRAM/1
  delay/1 -> split_into_int_and_frac_parts/1(delay)
  delayMatch1/1 -> integer delay DPRAM/2
  write address generator/1 -> delayMatch1/1, delayMatch/1
  Constant2/1 -> delayMatch2/1
  Constant/1 -> delayMatch3/1
  delayMatch5/1 -> fractional delay DPRAM/2
  write address generator1/1 -> delayMatch5/1, delayMatch4/1
  Constant1/1 -> delayMatch6/1
  split_into_int_and_frac_parts/1(integer_delay) -> read address generator/2(delay)
  CIC interpolation gain compensation/1 -> Data Type Conversion/1
  Downsample/1 -> PipelineRegister/1

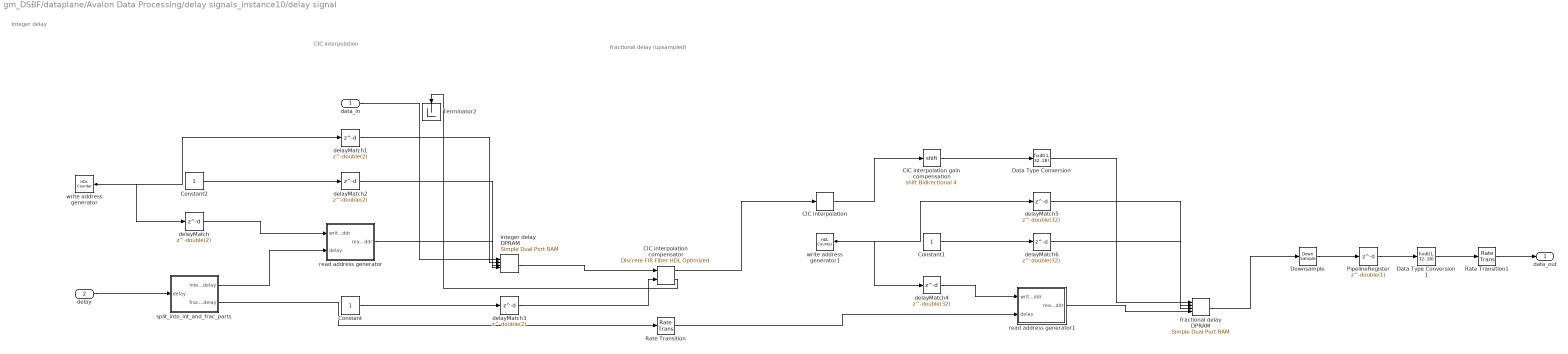
== system gm_DSBF/dataplane/Avalon Data Processing/delay signals_instance10/delay signal ==
  note: CIC interpolation
  note: Integer delay
  note: fractional delay (upsampled)
  data_in : Inport  OutDataTypeStr=fixdt(1, 32, 28)  PortDimensions=1  SampleTime=2.08333333333333e-05
  delay : Inport  Port=2  OutDataTypeStr=fixdt(1, 12, 6)  PortDimensions=1  SampleTime=2.08333333333333e-05
  CIC Interpolation : dspmlti4/CIC Interpolation  filtFrom=Filter object  filtobj=mp.cicInterpolator  ftype=Interpolator  R=mp.upsampleFactor  M=1  N=2  filterInternals=Full precision  BPS=[16 16 16 16]  FLPS=0  outputWordLength=32  outputFracLength=0  launchFVT=off  framing=Allow multirate processing  OutputFrames=off
      settings: SourceProductName=DSP System Toolbox  SourceProductBaseCode=DS
  CIC interpolation compensator : dsphdlfiltering/Discrete FIR Filter HDL Optimized  NumeratorSource=Property  Numerator=mp.cicInterpolatorCompensator.coeffs.Numerator  NumeratorPrototype=[]  FilterStructure=Direct form systolic  SerializationOption=Maximum number of multipliers  NumberOfCycles=2  NumberOfMultipliers=4  SimulateUsing=Code generation  roundingMode=Floor  overflowMode=off  CoefficientsDataTypeStr=fixdt(1,16)  CoefficientsMin=[]  CoefficientsMax=[]  OutputDataTypeStr=Inherit: Same word length as input  OutputMin=[]  OutputMax=[]  ResetInputPort=off  HDLGlobalReset=off
      settings: SourceProductName=DSP System Toolbox  SourceProductBaseCode=DS
  CIC interpolation gain compensation : ArithShift  BitShiftNumber=4  BinPtShiftNumber=double(0)
  Constant : Constant  OutDataTypeStr=boolean  SampleTime=-1
  Constant1 : Constant  OutDataTypeStr=boolean  SampleTime=-1
  Constant2 : Constant  OutDataTypeStr=boolean  SampleTime=-1
  Data Type Conversion : DataTypeConversion  OutDataTypeStr=fixdt(1, 32, 28)  SampleTime=1.30208333333333e-06
  Data Type Conversion1 : DataTypeConversion  OutDataTypeStr=fixdt(1, 32, 28)  SampleTime=2.08333333333333e-05
  Downsample : DownSample  N=double(16)  phase=double(0)  RateOptions=Allow multirate processing
  PipelineRegister : Delay  DelayLength=double(1)  InitialCondition=0  SampleTime=2.08333333333333e-05
  Rate Transition : RateTransition  InitialCondition=double(0)  OutPortSampleTimeOpt=Multiple of input port sample time  OutPortSampleTimeMultiple=1/16
  Rate Transition1 : RateTransition  InitialCondition=double(0)  OutPortSampleTimeOpt=Multiple of input port sample time  OutPortSampleTimeMultiple=1/2048
  Terminator2 : Terminator
  delayMatch{,1..3} (4 alike) : Delay  DelayLength=double(2)  InitialCondition=0  SampleTime=2.08333333333333e-05
  delayMatch4 : Delay  DelayLength=double(32)  InitialCondition=0  SampleTime=1.30208333333333e-06
  delayMatch5 : Delay  DelayLength=double(32)  InitialCondition=0  SampleTime=1.30208333333333e-06
  delayMatch6 : Delay  DelayLength=double(32)  InitialCondition=0  SampleTime=1.30208333333333e-06
  fractional delay DPRAM : hdlsllib/HDL RAMs/Simple Dual Port RAM  ram_size=mp.fractionalDelayAddrSize
      settings: SourceProductName=Simulink  SourceProductBaseCode=SL
  integer delay DPRAM : hdlsllib/HDL RAMs/Simple Dual Port RAM  ram_size=mp.integerDelayAddrSize
      settings: SourceProductName=Simulink  SourceProductBaseCode=SL
  read address generator : Subsystem
  read address generator1 : Subsystem
  split_into_int_and_frac_parts : Subsystem
  write address generator : hdlsllib/Sources/HDL Counter  CountType=Count limited  CountInit=double(0)  CountStep=double(1)  CountMax=double(63)  CountFromType=Initial value  CountFrom=double(0)  CountResetPort=off  CountLoadPort=off  CountEnbPort=off  CountDirPort=off  CountDataType=Unsigned  CountWordLen=6  CountFracLen=0  CountSampTime=2.08333333333333e-05
      settings: SourceProductName=Simulink
  write address generator1 : hdlsllib/Sources/HDL Counter  CountType=Count limited  CountInit=double(0)  CountStep=double(1)  CountMax=double(63)  CountFromType=Initial value  CountFrom=double(0)  CountResetPort=off  CountLoadPort=off  CountEnbPort=off  CountDirPort=off  CountDataType=Unsigned  CountWordLen=6  CountFracLen=0  CountSampTime=1.30208333333333e-06
      settings: SourceProductName=Simulink
  data_out : Outport  VectorParamsAs1DForOutWhenUnconnected=off
  wires:
  Downsample/1 -> PipelineRegister/1
  CIC interpolation gain compensation/1 -> Data Type Conversion/1
  split_into_int_and_frac_parts/1(integer_delay) -> read address generator/2(delay)
  Constant1/1 -> delayMatch6/1
  write address generator1/1 -> delayMatch4/1, delayMatch5/1
  delayMatch5/1 -> fractional delay DPRAM/2
  Constant/1 -> delayMatch3/1
  Constant2/1 -> delayMatch2/1
  write address generator/1 -> delayMatch/1, delayMatch1/1
  delayMatch1/1 -> integer delay DPRAM/2
  delay/1 -> split_into_int_and_frac_parts/1(delay)
  data_in/1 -> integer delay DPRAM/1
  delayMatch3/1 -> CIC interpolation compensator/2
  delayMatch6/1 -> fractional delay DPRAM/3
  delayMatch2/1 -> integer delay DPRAM/3
  Data Type Conversion/1 -> fractional delay DPRAM/1
  Data Type Conversion1/1 -> Rate Transition1/1
  split_into_int_and_frac_parts/2(fractional_delay) -> Rate Transition/1
  read address generator/1(read_addr) -> integer delay DPRAM/4
  read address generator1/1(read_addr) -> fractional delay DPRAM/4
  CIC Interpolation/1 -> CIC interpolation gain compensation/1
  CIC interpolation compensator/2 -> Terminator2/1
  CIC interpolation compensator/1 -> CIC Interpolation/1
  PipelineRegister/1 -> Data Type Conversion1/1
  Rate Transition/1 -> read address generator1/2(delay)
  Rate Transition1/1 -> data_out/1
  fractional delay DPRAM/1 -> Downsample/1
  integer delay DPRAM/1 -> CIC interpolation compensator/1
  delayMatch/1 -> read address generator/1(write_addr)
  delayMatch4/1 -> read address generator1/1(write_addr)
